simulink model "ramses_test"  (R2018b)
settings: Solver=FixedStepAuto  StartTime=0.0  StopTime=240  FixedStep=0.5  RelTol=1e-3
settings Model: Creator=apetros  LastModifiedBy=eenpar
settings DebuggingCC: AlgebraicLoopMsg=none  LibraryContextMissingDiagnostic=none
settings SFSimCC: SimUseLocalCustomCode=off
settings RTWCC: RTWUseLocalCustomCode=off

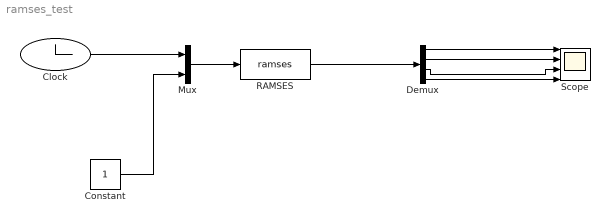
== system ramses_test ==
  Clock : Clock
  Constant : Constant
  Demux : Demux
  Mux : Mux  Inputs=2
  RAMSES : MATLABFcn  InitFcn=ramses_init  MATLABFcn=ramses
  Scope : Scope  NumInputPorts=4
  wires:
  RAMSES/1 -> Demux/1
  Demux/1 -> Scope/1
  Demux/2 -> Scope/2
  Demux/3 -> Scope/3
  Clock/1 -> Mux/1
  Mux/1 -> RAMSES/1
  Demux/4 -> Scope/4
  Constant/1 -> Mux/2
